simulink model "es1_sim"  (Simulink 7.5)
settings: Solver=ode45  StartTime=0.0  StopTime=5  RelTol=1e-3
libraries: simulink x1
settings Model: Creator=76936  LastModifiedBy=76936

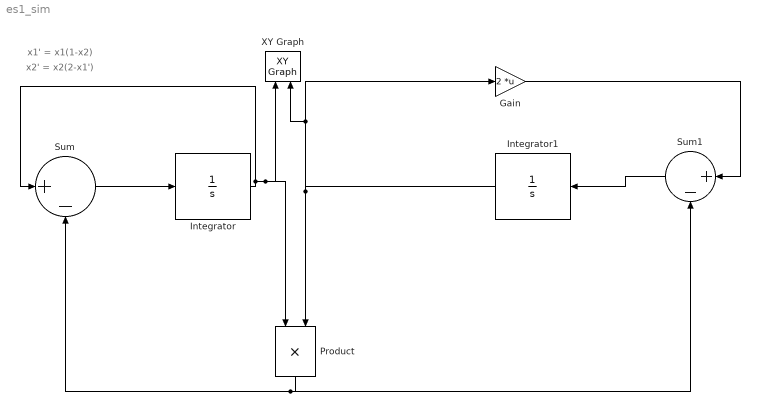
== system es1_sim ==
  note: x1' = x1(1-x2)
  note: x2' = x2(2-x1')
  Gain : Gain  Gain=2  Multiplication=Matrix(K*u)  ParameterDataType=fixdt(1, 16)  ParameterScaling=2^0  OutDataType=fixdt(1, 16)  OutScaling=2^0
  Integrator : Integrator  InitialCondition=10
  Integrator1 : Integrator  InitialCondition=10
  Product : Product  OutDataType=fixdt(1, 16)  OutScaling=2^0  RndMeth=Zero
  Sum : Sum  Inputs=|+-  OutDataType=fixdt(1, 16)  OutScaling=2^0
  Sum1 : Sum  Inputs=|+-  OutDataType=fixdt(1, 16)  OutScaling=2^0
  XY Graph : simulink/Sinks/XY Graph  SystemSampleTime=-1  xmin=-20  xmax=20  ymin=-20  ymax=20  st=-1
  wires:
  Integrator/1 -> Sum/1, Product/1, XY Graph/1
  Integrator1/1 -> Product/2, Gain/1, XY Graph/2
  Product/1 -> Sum/2, Sum1/2
  Sum/1 -> Integrator/1
  Gain/1 -> Sum1/1
  Sum1/1 -> Integrator1/1
